simulink model "SystemModel"  (R2017a)
settings: Solver=VariableStepAuto  StartTime=0.0  StopTime=10  RelTol=1e-3
values from neighbouring files (symbols this model uses):
  Amp0d = 1    [System.m]
  Amp0n = 1    [System.m]
  Amp1d = 1    [System.m]
  Amp1n = 1    [System.m]
  Elec0d = [M0(TermL),M0(TermR)]    [System.m]
  Elec0n = [1]    [System.m]
  Elec1d = [M1(TermL),M1(TermR)]    [System.m]
  Elec1n = [1]    [System.m]
  Mech0d = [M0(RotJ) + SysJ0, Dyan_Fric0]    [System.m]
  Mech0n = [1]    [System.m]
  Mech1d = [M1(RotJ) + SysJ1, Dyan_Fric1]    [System.m]
  Mech1n = [1]    [System.m]
  NomCurr0 = M0(NomCurr)    [System.m]
  NomCurr1 = M1(NomCurr)    [System.m]
  Sens0 = 1    [System.m]
  Sens1 = 1    [System.m]
  SpdCon0 = M0(SpdK)    [System.m]
  SpdCon1 = M1(SpdK)    [System.m]
  StallCurr0 = M0(StallCurr)    [System.m]
  StallCurr1 = M1(StallCurr)    [System.m]
  TCon0 = M0(TorqueK)    [System.m]
  TCon1 = M1(TorqueK)    [System.m]
libraries: simulink x13
settings Model: Creator=Matthew  LastModifiedBy=Matthew

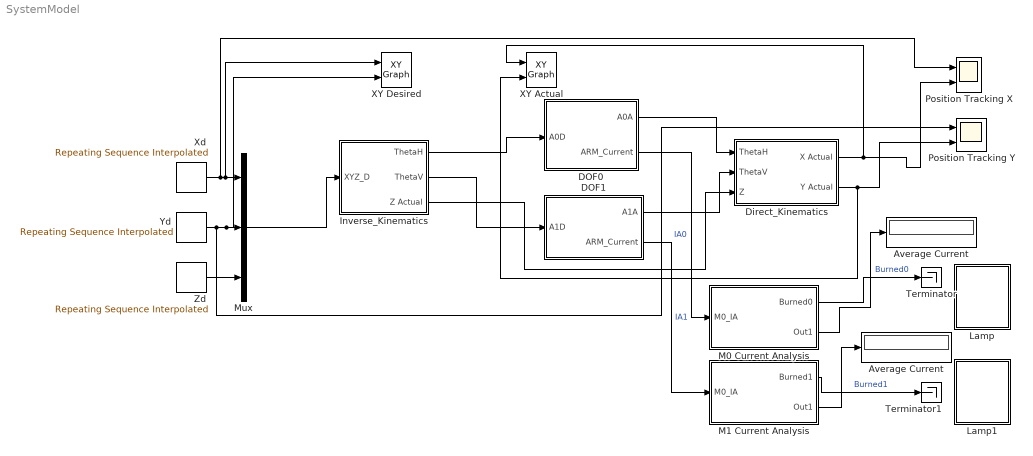
== system SystemModel ==
  Average Current : Display
      settings: Decimation=3
  "Average Current " : Display
      settings: Decimation=3
  DOF0 : Subsystem
  DOF1 : Subsystem
  Direct_Kinematics : Subsystem
  "Inverse_Kinematics " : Subsystem
  Lamp : Subsystem  DialogController=hmiCreateDDGDialog  IsWebBlock=on  mask(MWDashboardBlock){webBlockId=9779a3d2-3bef-4568-b22c-5c726568c4e1, webBlockType=lamp, ShowInLibBrowser=on, ShowInitialText=on, HMISrcModelName=SystemModel}
      mask prompts: webBlockType "WebBlock Type"; HMISrcModelName "Source Model"
      mask help: SimulinkHMI:dialogs:LampDialogDesc
      mask Help: helpview([docroot '/mapfiles/simulink.map'], 'hmi_lamp')
      mask Display:
      | if strcmp(get_param(bdroot(gcb),'BlockDiagramType'), 'library')
      |     image([(matlabroot) '/toolbox/simulink/hmi/icons/Lamp.png']);
      | end
  Lamp1 : Subsystem  DialogController=hmiCreateDDGDialog  IsWebBlock=on  mask(MWDashboardBlock){webBlockId=6168aa36-7ed6-404b-a80d-e64d244c71c2, webBlockType=lamp, ShowInLibBrowser=on, ShowInitialText=on, HMISrcModelName=SystemModel}
      mask prompts: webBlockType "WebBlock Type"; HMISrcModelName "Source Model"
      mask help: SimulinkHMI:dialogs:LampDialogDesc
      mask Help: helpview([docroot '/mapfiles/simulink.map'], 'hmi_lamp')
      mask Display:
      | if strcmp(get_param(bdroot(gcb),'BlockDiagramType'), 'library')
      |     image([(matlabroot) '/toolbox/simulink/hmi/icons/Lamp.png']);
      | end
  "M0 Current Analysis " : Subsystem
  "M1 Current Analysis " : Subsystem
  Mux : Mux  Inputs=3
  Position Tracking X : Scope  NumInputPorts=2
  "Position Tracking Y " : Scope  NumInputPorts=2
  Terminator : Terminator
  Terminator1 : Terminator
  "XY Actual " : simulink/Sinks/XY Graph  xmin=-12  xmax=12  ymin=-12  ymax=12  st=0.1
  "XY Desired " : simulink/Sinks/XY Graph  xmin=-12  xmax=12  ymin=-12  ymax=12  st=0.1
  "Xd " : simulink/Sources/Repeating Sequence Interpolated  OutValues=Xd  TimeValues=Time  LookUpMeth=Interpolation-Use End Values  tsamp=SampleTime  OutMin=[]  OutMax=[]  OutDataTypeStr=double  OutputDataTypeScalingMode=double  OutDataType=fixdt(0,8)  OutScaling=2^-10
  Yd : simulink/Sources/Repeating Sequence Interpolated  OutValues=Yd  TimeValues=Time  LookUpMeth=Interpolation-Use End Values  tsamp=SampleTime  OutMin=[]  OutMax=[]  OutDataTypeStr=double  OutputDataTypeScalingMode=double  OutDataType=fixdt(0,8)  OutScaling=2^-10
  "Zd " : simulink/Sources/Repeating Sequence Interpolated  OutValues=Zd  TimeValues=Time  LookUpMeth=Interpolation-Use End Values  tsamp=SampleTime  OutMin=[]  OutMax=[]  OutDataTypeStr=double  OutputDataTypeScalingMode=double  OutDataType=fixdt(0,8)  OutScaling=2^-10
  wires:
  Mux/1 -> "Inverse_Kinematics "/1(XYZ_D)
  "Inverse_Kinematics "/2(ThetaV) -> DOF1/1(A1D)
  DOF0/1(A0A) -> Direct_Kinematics/1("ThetaH ")
  DOF1/1("A1A ") -> Direct_Kinematics/2(ThetaV)
  Direct_Kinematics/1("X Actual ") -> "XY Actual "/1, Position Tracking X/2
  Direct_Kinematics/2(Y Actual) -> "Position Tracking Y "/2, "XY Actual "/2
  DOF0/2("ARM_Current ") -> "M0 Current Analysis "/1(M0_IA)  "IA0"
  DOF1/2("ARM_Current ") -> "M1 Current Analysis "/1(M0_IA)  "IA1"
  "M0 Current Analysis "/1("Burned0 ") -> Terminator/1  "Burned0"
  "M1 Current Analysis "/1("Burned1 ") -> Terminator1/1  "Burned1"
  "Inverse_Kinematics "/1(ThetaH) -> DOF0/1(A0D)
  "Inverse_Kinematics "/3("Z Actual ") -> Direct_Kinematics/3("Z ")
  "M0 Current Analysis "/2(Out1) -> Average Current/1
  "M1 Current Analysis "/2(Out1) -> "Average Current "/1
  "Xd "/1 -> Position Tracking X/1, "XY Desired "/1, Mux/1
  Yd/1 -> "Position Tracking Y "/1, "XY Desired "/2, Mux/2
  "Zd "/1 -> Mux/3

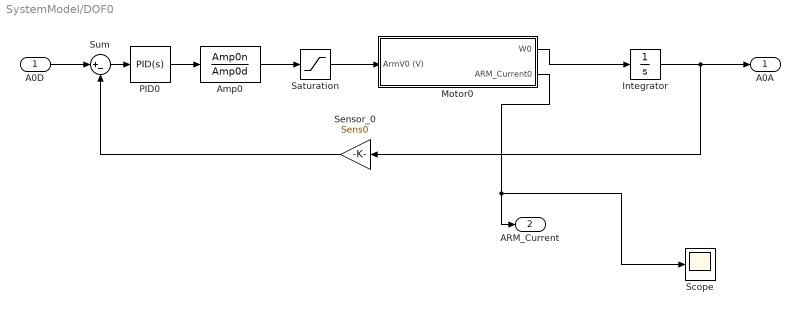
== system SystemModel/DOF0 ==
  A0D : Inport
  "Amp0 " : TransferFcn  Numerator=Amp0n  Denominator=Amp0d
  Integrator : Integrator
  "Motor0 " : Subsystem
  "PID0 " : simulink/Continuous/PID Controller  Controller=PID  TimeDomain=Continuous-time  SampleTime=-1  IntegratorMethod=Forward Euler  FilterMethod=Forward Euler  Form=Parallel  UseFilter=on  ControllerParametersSource=internal  P=4.43200114507061  I=26.5426511653012  D=0.120281260642519  N=35110.2640373981  InitialConditionSource=internal  InitialConditionForIntegrator=0  InitialConditionForFilter=0  ExternalReset=none  LimitOutput=off  UpperSaturationLimit=inf  LowerSaturationLimit=-inf  LinearizeAsGain=on  AntiWindupMode=none  Kb=1  TrackingMode=off  Kt=1  PParamMin=[]  PParamMax=[]  IParamMin=[]  IParamMax=[]  DParamMin=[]  DParamMax=[]  NParamMin=[]  NParamMax=[]  KbParamMin=[]  KbParamMax=[]  KtParamMin=[]  KtParamMax=[]  POutMin=[]  POutMax=[]  IOutMin=[]  IOutMax=[]  DOutMin=[]  DOutMax=[]  NOutMin=[]  NOutMax=[]  KbOutMin=[]  KbOutMax=[]  KtOutMin=[]  KtOutMax=[]  IntegratorOutMin=[]  IntegratorOutMax=[]  FilterOutMin=[]  FilterOutMax=[]  SumOutMin=[]  SumOutMax=[]  SumI1OutMin=[]  SumI1OutMax=[]  SumI2OutMin=[]  SumI2OutMax=[]  SumI3OutMin=[]  SumI3OutMax=[]  SumDOutMin=[]  SumDOutMax=[]  SaturationOutMin=[]  SaturationOutMax=[]  IntegratorContinuousStateAttributes=''  IntegratorStateMustResolveToSignalObject=off  IntegratorRTWStateStorageClass=Auto  FilterContinuousStateAttributes=''  FilterStateMustResolveToSignalObject=off  FilterRTWStateStorageClass=Auto  DifferentiatorICPrevScaledInput=0  DifferentiatorOutMin=[]  DifferentiatorOutMax=[]  InitialConditionSetting=State (most efficient)
  Saturation : Saturate  UpperLimit=20  LowerLimit=-20
  Scope : Scope
  Sensor_0 : Gain  Gain=Sens0
  Sum : Sum  Inputs=|+-
  A0A : Outport
  "ARM_Current " : Outport  Port=2
  wires:
  Integrator/1 -> A0A/1, Sensor_0/1
  "Motor0 "/1("W0 ") -> Integrator/1
  Sum/1 -> "PID0 "/1
  Sensor_0/1 -> Sum/2
  A0D/1 -> Sum/1
  "Motor0 "/2("ARM_Current0 ") -> Scope/1, "ARM_Current "/1
  "PID0 "/1 -> "Amp0 "/1
  Saturation/1 -> "Motor0 "/1(ArmV0 (V))
  "Amp0 "/1 -> Saturation/1

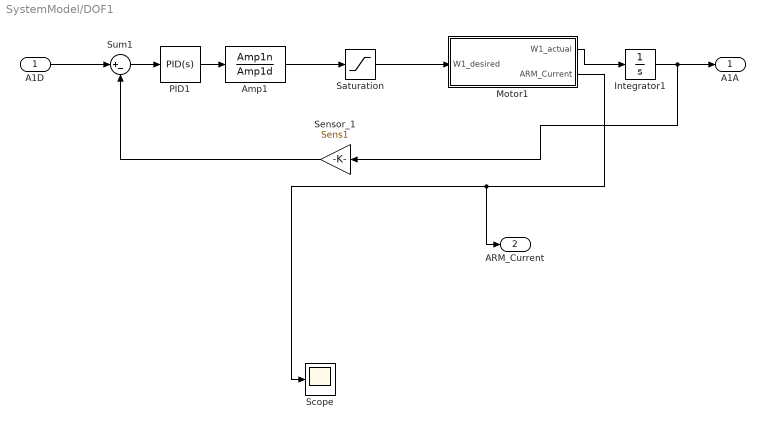
== system SystemModel/DOF1 ==
  A1D : Inport
  "Amp1 " : TransferFcn  Numerator=Amp1n  Denominator=Amp1d
  Integrator1 : Integrator
  "Motor1 " : Subsystem
  "PID1 " : simulink/Continuous/PID Controller  Controller=PID  TimeDomain=Continuous-time  SampleTime=-1  IntegratorMethod=Forward Euler  FilterMethod=Forward Euler  Form=Parallel  UseFilter=on  ControllerParametersSource=internal  P=7.51859884189587  I=27.6504163799551  D=0.183682887852162  N=53357.4410558719  InitialConditionSource=internal  InitialConditionForIntegrator=0  InitialConditionForFilter=0  ExternalReset=none  LimitOutput=off  UpperSaturationLimit=inf  LowerSaturationLimit=-inf  LinearizeAsGain=on  AntiWindupMode=none  Kb=1  TrackingMode=off  Kt=1  PParamMin=[]  PParamMax=[]  IParamMin=[]  IParamMax=[]  DParamMin=[]  DParamMax=[]  NParamMin=[]  NParamMax=[]  KbParamMin=[]  KbParamMax=[]  KtParamMin=[]  KtParamMax=[]  POutMin=[]  POutMax=[]  IOutMin=[]  IOutMax=[]  DOutMin=[]  DOutMax=[]  NOutMin=[]  NOutMax=[]  KbOutMin=[]  KbOutMax=[]  KtOutMin=[]  KtOutMax=[]  IntegratorOutMin=[]  IntegratorOutMax=[]  FilterOutMin=[]  FilterOutMax=[]  SumOutMin=[]  SumOutMax=[]  SumI1OutMin=[]  SumI1OutMax=[]  SumI2OutMin=[]  SumI2OutMax=[]  SumI3OutMin=[]  SumI3OutMax=[]  SumDOutMin=[]  SumDOutMax=[]  SaturationOutMin=[]  SaturationOutMax=[]  IntegratorContinuousStateAttributes=''  IntegratorStateMustResolveToSignalObject=off  IntegratorRTWStateStorageClass=Auto  FilterContinuousStateAttributes=''  FilterStateMustResolveToSignalObject=off  FilterRTWStateStorageClass=Auto  DifferentiatorICPrevScaledInput=0  DifferentiatorOutMin=[]  DifferentiatorOutMax=[]  InitialConditionSetting=State (most efficient)
  Saturation : Saturate  UpperLimit=20  LowerLimit=-20
  Scope : Scope
  Sensor_1 : Gain  Gain=Sens1
  Sum1 : Sum  Inputs=|+-
  "A1A " : Outport
  "ARM_Current " : Outport  Port=2
  wires:
  Sensor_1/1 -> Sum1/2
  Sum1/1 -> "PID1 "/1
  Integrator1/1 -> "A1A "/1, Sensor_1/1
  A1D/1 -> Sum1/1
  "Motor1 "/1("W1_actual ") -> Integrator1/1
  "Motor1 "/2("ARM_Current ") -> Scope/1, "ARM_Current "/1
  "PID1 "/1 -> "Amp1 "/1
  "Amp1 "/1 -> Saturation/1
  Saturation/1 -> "Motor1 "/1(W1_desired)

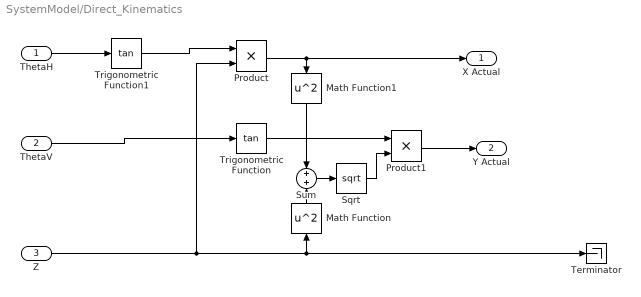
== system SystemModel/Direct_Kinematics ==
  "ThetaH " : Inport
  ThetaV : Inport  Port=2
  "Z " : Inport  Port=3
  Math Function : Math  Operator=square  SaturateOnIntegerOverflow=on
  Math Function1 : Math  Operator=square  SaturateOnIntegerOverflow=on
  Product : Product
  Product1 : Product
  Sqrt : Sqrt  SaturateOnIntegerOverflow=on
  Sum : Sum  Inputs=+|+
  Terminator : Terminator
  Trigonometric Function : Trigonometry  Operator=tan
  Trigonometric Function1 : Trigonometry  Operator=tan
  "X Actual " : Outport
  Y Actual : Outport  Port=2
  wires:
  "Z "/1 -> Product/2, Math Function/1, Terminator/1
  ThetaV/1 -> Trigonometric Function/1
  "ThetaH "/1 -> Trigonometric Function1/1
  Trigonometric Function1/1 -> Product/1
  Product/1 -> "X Actual "/1, Math Function1/1
  Math Function/1 -> Sum/2
  Math Function1/1 -> Sum/1
  Sum/1 -> Sqrt/1
  Product1/1 -> Y Actual/1
  Trigonometric Function/1 -> Product1/1
  Sqrt/1 -> Product1/2

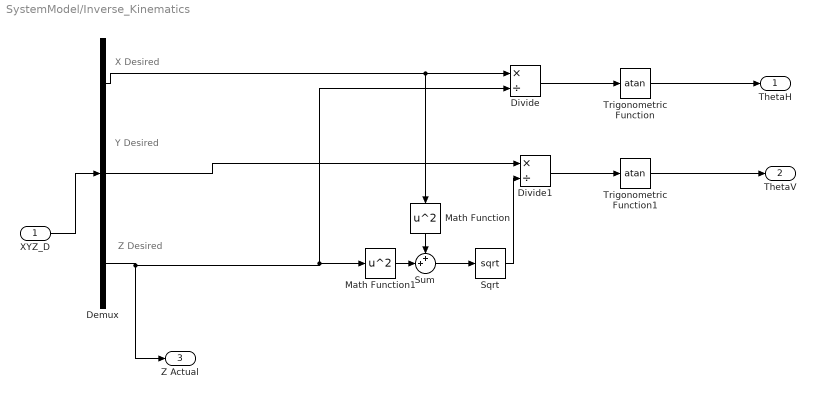
== system SystemModel/Inverse_Kinematics  ==
  note: Z Desired
  note: Y Desired
  note: X Desired
  XYZ_D : Inport
  Demux : Demux  Outputs=3
  Divide : Product  Inputs=*/
  Divide1 : Product  Inputs=*/
  Math Function : Math  Operator=square  SaturateOnIntegerOverflow=on
  Math Function1 : Math  Operator=square  SaturateOnIntegerOverflow=on
  Sqrt : Sqrt  SaturateOnIntegerOverflow=on
  Sum : Sum  Inputs=++|
  Trigonometric Function : Trigonometry  Operator=atan
  Trigonometric Function1 : Trigonometry  Operator=atan
  ThetaH : Outport
  ThetaV : Outport  Port=2
  "Z Actual " : Outport  Port=3
  wires:
  XYZ_D/1 -> Demux/1
  Demux/3 -> Math Function1/1, Divide/2, "Z Actual "/1
  Trigonometric Function/1 -> ThetaH/1
  Divide/1 -> Trigonometric Function/1
  Demux/1 -> Math Function/1, Divide/1
  Math Function/1 -> Sum/1
  Math Function1/1 -> Sum/2
  Sum/1 -> Sqrt/1
  Sqrt/1 -> Divide1/2
  Demux/2 -> Divide1/1
  Divide1/1 -> Trigonometric Function1/1
  Trigonometric Function1/1 -> ThetaV/1

== system SystemModel/Lamp ==

== system SystemModel/Lamp1 ==

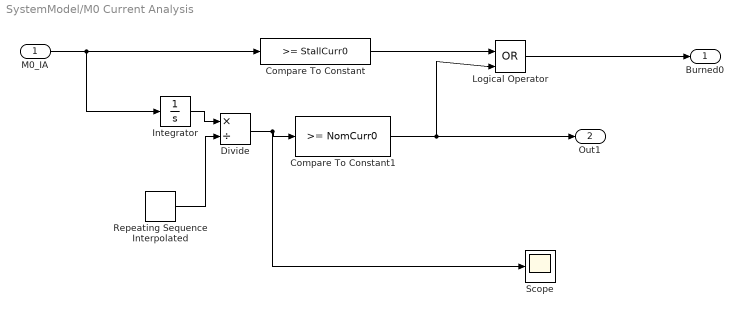
== system SystemModel/M0 Current Analysis  ==
  M0_IA : Inport
  Compare To Constant : simulink/Logic and Bit Operations/Compare To Constant  relop=>=  const=StallCurr0  OutDataTypeStr=boolean
  Compare To Constant1 : simulink/Logic and Bit Operations/Compare To Constant  relop=>=  const=NomCurr0  OutDataTypeStr=boolean
  Divide : Product  Inputs=*/
  Integrator : Integrator
  Logical Operator : Logic  Operator=OR  IconShape=distinctive  AllPortsSameDT=off  OutDataTypeStr=boolean
  Repeating Sequence Interpolated : simulink/Sources/Repeating Sequence Interpolated  OutValues=Time  TimeValues=Time  LookUpMeth=Interpolation-Use End Values  tsamp=0.01  OutMin=[]  OutMax=[]  OutDataTypeStr=double  OutputDataTypeScalingMode=double  OutDataType=fixdt(0,8)  OutScaling=2^-10
  Scope : Scope
  "Burned0 " : Outport
  Out1 : Outport  Port=2
  wires:
  Repeating Sequence Interpolated/1 -> Divide/2
  M0_IA/1 -> Compare To Constant/1, Integrator/1
  Integrator/1 -> Divide/1
  Divide/1 -> Scope/1, Compare To Constant1/1
  Compare To Constant1/1 -> Out1/1, Logical Operator/2
  Compare To Constant/1 -> Logical Operator/1
  Logical Operator/1 -> "Burned0 "/1

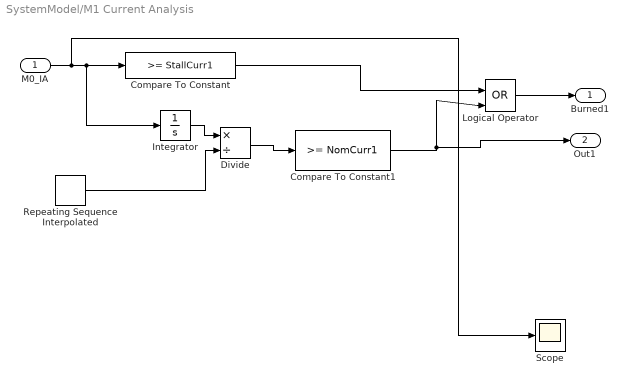
== system SystemModel/M1 Current Analysis  ==
  M0_IA : Inport
  Compare To Constant : simulink/Logic and Bit Operations/Compare To Constant  relop=>=  const=StallCurr1  OutDataTypeStr=boolean
  Compare To Constant1 : simulink/Logic and Bit Operations/Compare To Constant  relop=>=  const=NomCurr1  OutDataTypeStr=boolean
  Divide : Product  Inputs=*/
  Integrator : Integrator
  Logical Operator : Logic  Operator=OR  IconShape=distinctive  AllPortsSameDT=off  OutDataTypeStr=boolean
  Repeating Sequence Interpolated : simulink/Sources/Repeating Sequence Interpolated  OutValues=Time  TimeValues=Time  LookUpMeth=Interpolation-Use End Values  tsamp=0.01  OutMin=[]  OutMax=[]  OutDataTypeStr=double  OutputDataTypeScalingMode=double  OutDataType=fixdt(0,8)  OutScaling=2^-10
  Scope : Scope
  "Burned1 " : Outport
  Out1 : Outport  Port=2
  wires:
  Repeating Sequence Interpolated/1 -> Divide/2
  M0_IA/1 -> Scope/1, Integrator/1, Compare To Constant/1
  Integrator/1 -> Divide/1
  Divide/1 -> Compare To Constant1/1
  Compare To Constant1/1 -> Out1/1, Logical Operator/2
  Compare To Constant/1 -> Logical Operator/1
  Logical Operator/1 -> "Burned1 "/1

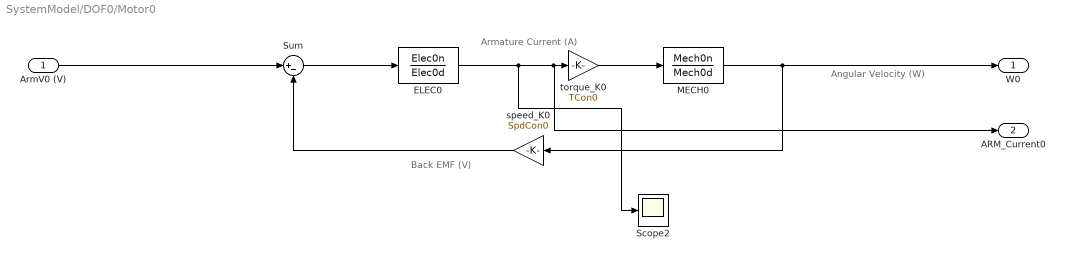
== system SystemModel/DOF0/Motor0  ==
  note: Back EMF
      | (V)
  note: Armature Current (A)
  note: Angular Velocity (W)
  ArmV0 (V) : Inport
  "ELEC0 " : TransferFcn  Numerator=Elec0n  Denominator=Elec0d
  "MECH0 " : TransferFcn  Numerator=Mech0n  Denominator=Mech0d
  Scope2 : Scope
  Sum : Sum  Inputs=|+-
  speed_K0 : Gain  Gain=SpdCon0
  torque_K0 : Gain  Gain=TCon0
  "W0 " : Outport
  "ARM_Current0 " : Outport  Port=2
  wires:
  ArmV0 (V)/1 -> Sum/1
  speed_K0/1 -> Sum/2
  "MECH0 "/1 -> "W0 "/1, speed_K0/1
  "ELEC0 "/1 -> Scope2/1, torque_K0/1, "ARM_Current0 "/1
  torque_K0/1 -> "MECH0 "/1
  Sum/1 -> "ELEC0 "/1

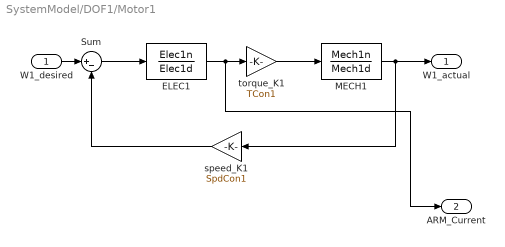
== system SystemModel/DOF1/Motor1  ==
  W1_desired : Inport
  "ELEC1 " : TransferFcn  Numerator=Elec1n  Denominator=Elec1d
  "MECH1 " : TransferFcn  Numerator=Mech1n  Denominator=Mech1d
  Sum : Sum  Inputs=|+-
  speed_K1 : Gain  Gain=SpdCon1
  "torque_K1 " : Gain  Gain=TCon1
  "W1_actual " : Outport
  "ARM_Current " : Outport  Port=2
  wires:
  Sum/1 -> "ELEC1 "/1
  W1_desired/1 -> Sum/1
  speed_K1/1 -> Sum/2
  "MECH1 "/1 -> "W1_actual "/1, speed_K1/1
  "ELEC1 "/1 -> "ARM_Current "/1, "torque_K1 "/1
  "torque_K1 "/1 -> "MECH1 "/1
